simulink model "IncompleetProgram"  (R2022a)
settings: Solver=VariableStepAuto  StartTime=0.0  StopTime=10.0  RelTol=1e-3
libraries: vexarmcortexlib x16, RoboticsPlayground x1
settings Model: Creator=impre  LastModifiedBy=impre

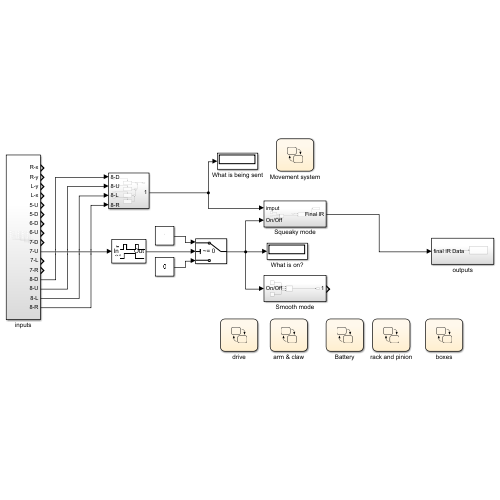
[thumbnail: Simulink's stored preview of the top-level diagram]
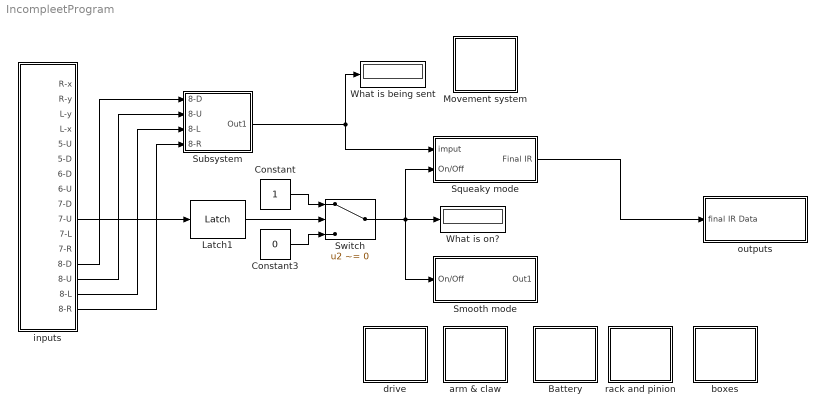
== system IncompleetProgram ==
  Battery : Stateflow chart  TreatAsAtomicUnit=on
  Constant : Constant
  Constant3 : Constant  Value=0
  Latch1 : RoboticsPlayground/Utilities and Hardware/Latch  SystemSampleTime=-1  VariantActivationTime=update diagram  Latency=0  AutoFrameSizeCalculation=off
      settings: SourceProductName=Robotics Playground
  Movement system : Stateflow chart  TreatAsAtomicUnit=on
  Smooth mode : Subsystem
  Squeaky mode : Subsystem
  Subsystem : Subsystem
  Switch : Switch  Criteria=u2 ~= 0  SaturateOnIntegerOverflow=off  InputSameDT=off
  What is being sent : Display
  What is on? : Display
  arm & claw : Stateflow chart  TreatAsAtomicUnit=on
  boxes : Stateflow chart  TreatAsAtomicUnit=on
  drive : Stateflow chart  TreatAsAtomicUnit=on
  inputs : Subsystem
  outputs : Subsystem
  rack and pinion : Stateflow chart  TreatAsAtomicUnit=on
  wires:
  Squeaky mode/1(Final IR) -> outputs/1(final IR Data)
  Constant/1 -> Switch/1
  Latch1/1 -> Switch/2
  Constant3/1 -> Switch/3
  Switch/1 -> What is on?/1, Smooth mode/1(On/Off), Squeaky mode/2(On/Off)
  inputs/10(7-U) -> Latch1/1
  inputs/16(8-R) -> Subsystem/4(8-R)
  inputs/15(8-L) -> Subsystem/3(8-L)
  inputs/14(8-U) -> Subsystem/2(8-U)
  inputs/13(8-D) -> Subsystem/1(8-D)
  Subsystem/1(Out1) -> What is being sent/1, Squeaky mode/1(imput)

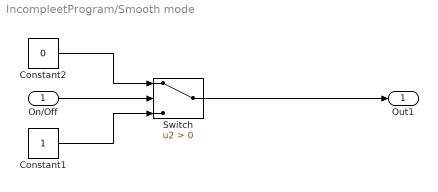
== system IncompleetProgram/Smooth mode ==
  On/Off : Inport
  Constant1 : Constant
  Constant2 : Constant  Value=0
  Switch : Switch  Criteria=u2 > Threshold  SaturateOnIntegerOverflow=off  InputSameDT=off
  Out1 : Outport
  wires:
  Switch/1 -> Out1/1
  Constant2/1 -> Switch/1
  On/Off/1 -> Switch/2
  Constant1/1 -> Switch/3

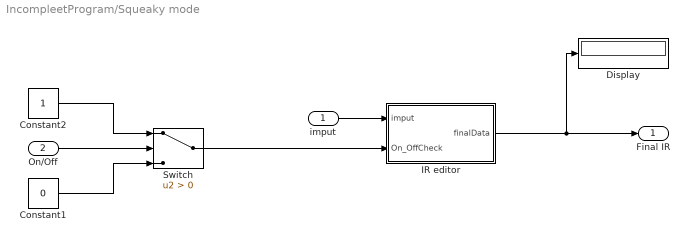
== system IncompleetProgram/Squeaky mode ==
  imput : Inport
  On/Off : Inport  Port=2
  Constant1 : Constant  Value=0
  Constant2 : Constant
  Display : Display
  IR editor : Stateflow chart  TreatAsAtomicUnit=on
  Switch : Switch  Criteria=u2 > Threshold  SaturateOnIntegerOverflow=off  InputSameDT=off
  Final IR : Outport
  wires:
  IR editor/1(finalData) -> Display/1, Final IR/1
  On/Off/1 -> Switch/2
  Constant1/1 -> Switch/3
  Constant2/1 -> Switch/1
  Switch/1 -> IR editor/2(On_OffCheck)
  imput/1 -> IR editor/1(imput)

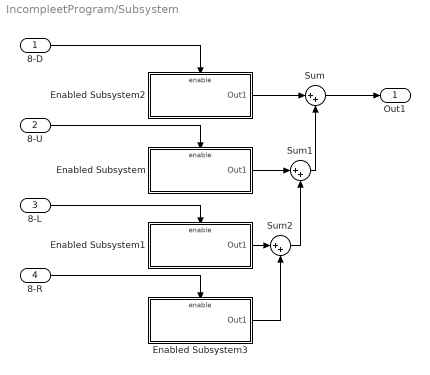
== system IncompleetProgram/Subsystem ==
  8-D : Inport
  8-U : Inport  Port=2
  8-L : Inport  Port=3
  8-R : Inport  Port=4
  Enabled Subsystem : Subsystem  TreatAsAtomicUnit=on
  Enabled Subsystem1 : Subsystem  TreatAsAtomicUnit=on
  Enabled Subsystem2 : Subsystem  TreatAsAtomicUnit=on
  Enabled Subsystem3 : Subsystem  TreatAsAtomicUnit=on
  Sum : Sum  Inputs=|++
  Sum1 : Sum  Inputs=|++
  Sum2 : Sum  Inputs=|++
  Out1 : Outport
  wires:
  8-D/1 -> Enabled Subsystem2/Enable
  8-U/1 -> Enabled Subsystem/Enable
  8-L/1 -> Enabled Subsystem1/Enable
  8-R/1 -> Enabled Subsystem3/Enable
  Enabled Subsystem2/1(Out1) -> Sum/1
  Sum/1 -> Out1/1
  Enabled Subsystem/1(Out1) -> Sum1/1
  Sum1/1 -> Sum/2
  Enabled Subsystem1/1(Out1) -> Sum2/1
  Sum2/1 -> Sum1/2
  Enabled Subsystem3/1(Out1) -> Sum2/2

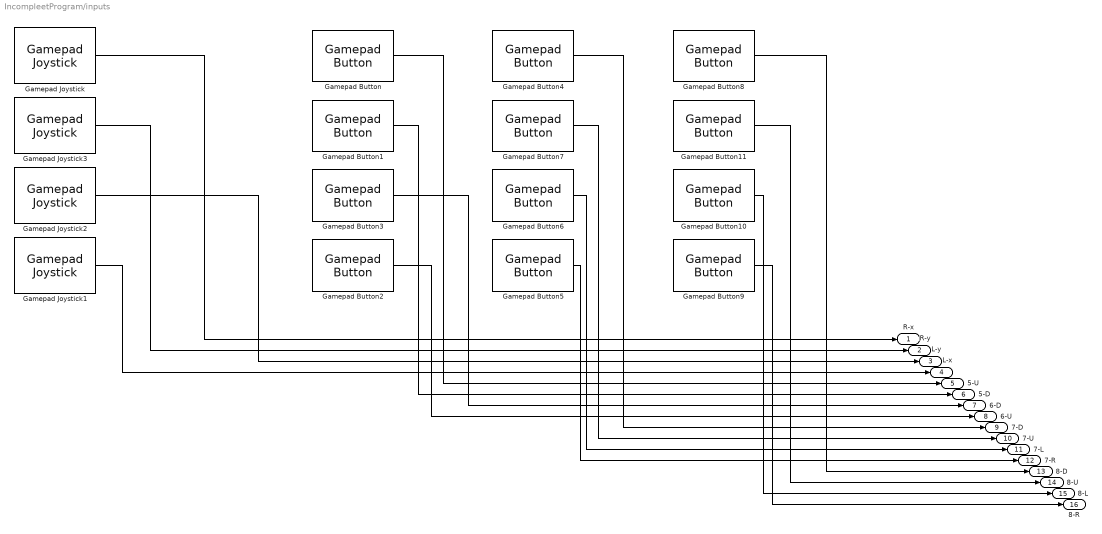
== system IncompleetProgram/inputs ==
  Gamepad Button : vexarmcortexlib/Gamepad/Gamepad Button  joystick=1  chan=5  button56=Up  button78=Down  SimulationIn=off  SampleTime=0.02
      settings: SourceProductBaseCode=EC_VEX_MICRO
  Gamepad Button1 : vexarmcortexlib/Gamepad/Gamepad Button  joystick=1  chan=5  button56=Down  button78=Down  SimulationIn=off  SampleTime=0.02
      settings: SourceProductBaseCode=EC_VEX_MICRO
  Gamepad Button10 : vexarmcortexlib/Gamepad/Gamepad Button  joystick=1  chan=8  button56=Up  button78=Left  SimulationIn=off  SampleTime=0.02
      settings: SourceProductBaseCode=EC_VEX_MICRO
  Gamepad Button11 : vexarmcortexlib/Gamepad/Gamepad Button  joystick=1  chan=8  button56=Up  button78=Up  SimulationIn=off  SampleTime=0.02
      settings: SourceProductBaseCode=EC_VEX_MICRO
  Gamepad Button2 : vexarmcortexlib/Gamepad/Gamepad Button  joystick=1  chan=6  button56=Up  button78=Down  SimulationIn=off  SampleTime=0.02
      settings: SourceProductBaseCode=EC_VEX_MICRO
  Gamepad Button3 : vexarmcortexlib/Gamepad/Gamepad Button  joystick=1  chan=6  button56=Down  button78=Down  SimulationIn=off  SampleTime=0.02
      settings: SourceProductBaseCode=EC_VEX_MICRO
  Gamepad Button4 : vexarmcortexlib/Gamepad/Gamepad Button  joystick=1  chan=7  button56=Up  button78=Down  SimulationIn=off  SampleTime=0.02
      settings: SourceProductBaseCode=EC_VEX_MICRO
  Gamepad Button5 : vexarmcortexlib/Gamepad/Gamepad Button  joystick=1  chan=7  button56=Up  button78=Right  SimulationIn=off  SampleTime=0.02
      settings: SourceProductBaseCode=EC_VEX_MICRO
  Gamepad Button6 : vexarmcortexlib/Gamepad/Gamepad Button  joystick=1  chan=7  button56=Up  button78=Left  SimulationIn=off  SampleTime=0.02
      settings: SourceProductBaseCode=EC_VEX_MICRO
  Gamepad Button7 : vexarmcortexlib/Gamepad/Gamepad Button  joystick=1  chan=7  button56=Up  button78=Up  SimulationIn=off  SampleTime=0.02
      settings: SourceProductBaseCode=EC_VEX_MICRO
  Gamepad Button8 : vexarmcortexlib/Gamepad/Gamepad Button  joystick=1  chan=8  button56=Up  button78=Down  SimulationIn=off  SampleTime=0.02
      settings: SourceProductBaseCode=EC_VEX_MICRO
  Gamepad Button9 : vexarmcortexlib/Gamepad/Gamepad Button  joystick=1  chan=8  button56=Up  button78=Right  SimulationIn=off  SampleTime=0.02
      settings: SourceProductBaseCode=EC_VEX_MICRO
  Gamepad Joystick : vexarmcortexlib/Gamepad/Gamepad Joystick  joystick=1  chan=1  SimulationIn=off  SampleTime=0.02
      settings: SourceProductBaseCode=EC_VEX_MICRO
  Gamepad Joystick1 : vexarmcortexlib/Gamepad/Gamepad Joystick  joystick=1  chan=4  SimulationIn=off  SampleTime=0.02
      settings: SourceProductBaseCode=EC_VEX_MICRO
  Gamepad Joystick2 : vexarmcortexlib/Gamepad/Gamepad Joystick  joystick=1  chan=3  SimulationIn=off  SampleTime=0.02
      settings: SourceProductBaseCode=EC_VEX_MICRO
  Gamepad Joystick3 : vexarmcortexlib/Gamepad/Gamepad Joystick  joystick=1  chan=2  SimulationIn=off  SampleTime=0.02
      settings: SourceProductBaseCode=EC_VEX_MICRO
  R-x : Outport
  R-y : Outport  Port=2
  L-y : Outport  Port=3
  L-x : Outport  Port=4
  5-U : Outport  Port=5
  5-D : Outport  Port=6
  6-D : Outport  Port=7
  6-U : Outport  Port=8
  7-D : Outport  Port=9
  7-U : Outport  Port=10
  7-L : Outport  Port=11
  7-R : Outport  Port=12
  8-D : Outport  Port=13
  8-U : Outport  Port=14
  8-L : Outport  Port=15
  8-R : Outport  Port=16
  wires:
  Gamepad Joystick/1 -> R-x/1
  Gamepad Joystick3/1 -> R-y/1
  Gamepad Joystick2/1 -> L-y/1
  Gamepad Joystick1/1 -> L-x/1
  Gamepad Button/1 -> 5-U/1
  Gamepad Button1/1 -> 5-D/1
  Gamepad Button3/1 -> 6-D/1
  Gamepad Button2/1 -> 6-U/1
  Gamepad Button4/1 -> 7-D/1
  Gamepad Button7/1 -> 7-U/1
  Gamepad Button6/1 -> 7-L/1
  Gamepad Button5/1 -> 7-R/1
  Gamepad Button8/1 -> 8-D/1
  Gamepad Button11/1 -> 8-U/1
  Gamepad Button10/1 -> 8-L/1
  Gamepad Button9/1 -> 8-R/1

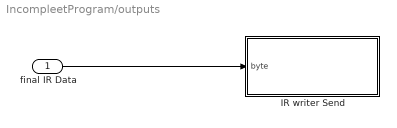
== system IncompleetProgram/outputs ==
  final IR Data : Inport
  IR writer Send : Subsystem
  wires:
  final IR Data/1 -> IR writer Send/1(byte)

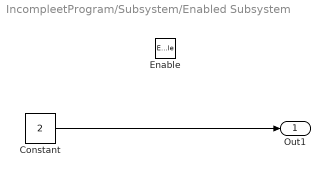
== system IncompleetProgram/Subsystem/Enabled Subsystem ==
  Enable : EnablePort
  Constant : Constant  Value=2
  Out1 : Outport
  wires:
  Constant/1 -> Out1/1

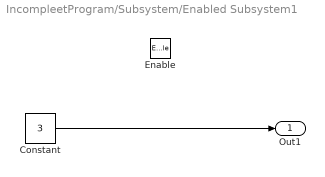
== system IncompleetProgram/Subsystem/Enabled Subsystem1 ==
  Enable : EnablePort
  Constant : Constant  Value=3
  Out1 : Outport
  wires:
  Constant/1 -> Out1/1

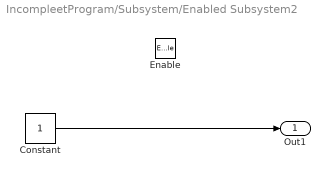
== system IncompleetProgram/Subsystem/Enabled Subsystem2 ==
  Enable : EnablePort
  Constant : Constant
  Out1 : Outport
  wires:
  Constant/1 -> Out1/1

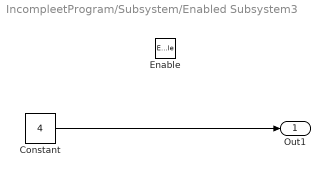
== system IncompleetProgram/Subsystem/Enabled Subsystem3 ==
  Enable : EnablePort
  Constant : Constant  Value=4
  Out1 : Outport
  wires:
  Constant/1 -> Out1/1

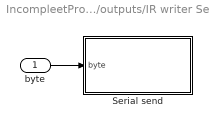
== system IncompleetProgram/outputs/IR writer Send ==
  byte : Inport  OutDataTypeStr=uint8  PortDimensions=[1 1]
  Serial send : MATLAB Function  TreatAsAtomicUnit=on
  wires:
  byte/1 -> Serial send/1(byte)

== stateflow chart IncompleetProgram/Movement system ==

== matlab function IncompleetProgram/outputs/IR writer Send/Serial send ==
  data: byte input
function fcn(byte)
% Serial send single byte
%#codegen

% Config
port = 'uart1';
baud = uint32(9600);

persistent isFirstRun

if coder.target('Rtw')
    coder.cinclude('API.h');
    coder.cinclude('string.h');
    file = coder.opaque('FILE *', port,'HeaderFile','API.h');

    if isempty(isFirstRun)
        % first time setup
        isFirstRun = false;

        flags = coder.opaque('uint16', 'SERIAL_8N1');
        coder.ceval('usartInit', file, baud, flags);
    end

    coder.ceval('fputc', byte, file);

end

end

== stateflow chart IncompleetProgram/drive ==

== stateflow chart IncompleetProgram/arm & claw ==

== stateflow chart IncompleetProgram/Battery ==

== stateflow chart IncompleetProgram/rack and pinion ==

== stateflow chart IncompleetProgram/boxes ==

== stateflow chart IncompleetProgram/Squeaky mode/IR editor ==
  state Test
    finalData = 0xF0;
    imput = 0;
  state CenterD
    finalData  = 0x66;
    imput = 0;
  state Initialize
    finalData =0x00;
  state CenterR
    finalData = 0xCC;
    imput = 0;
  state CenterL
    finalData = 0x5A;
    imput = 0;
  Initialize -> Test [order 1] : [imput == 1]
  Test -> Initialize
  Initialize -> CenterD [order 2] : [imput == 2]
  CenterD -> Initialize
  (default) -> Initialize : {On_OffCheck == 1}
  CenterR -> Initialize
  Initialize -> CenterL [order 3] : [imput == 4]
  CenterL -> Initialize
  Initialize -> CenterR [order 4] : [imput == 3]
  data: finalData output; imput input; On_OffCheck input
